simulink model "ACDCMG_woPV"  (R2022a)
settings: Solver=FixedStepAuto  StartTime=0.0  StopTime=0.2  FixedStep=Ts  MaxStep=1e-2  RelTol=1e-3
InitFcn:
  | Set_parameters_R2018
values from neighbouring files (symbols this model uses):
  D_invs = 0.05    [Set_parameters_R2018.m]
  dis11 = 3    [Set_parameters_R2018.m]
  dis14 = 2    [Set_parameters_R2018.m]
  dis2 = 0.2    [Set_parameters_R2018.m]
  dis3 = 0.15    [Set_parameters_R2018.m]
  dis4 = 0.4    [Set_parameters_R2018.m]
  dis5 = 0.4    [Set_parameters_R2018.m]
  dis6 = 0.4    [Set_parameters_R2018.m]
  dis8 = 2    [Set_parameters_R2018.m]
  Fnom = 60    [Set_parameters_R2018.m]
  H_invs = 6    [Set_parameters_R2018.m]
  max_min = 1    [Set_parameters_R2018.m]
  P_Load_3 = S_Load_3* PF_Load_3    (= 25500)    [Set_parameters_R2018.m]
  P_nom_inv = 3e3    (= 3000)    [Set_parameters_R2018.m]
  Pnom_T1 = 1.5e6    (= 1500000)    [Set_parameters_R2018.m]
  Pnom_T2 = 1.5e6    (= 1500000)    [Set_parameters_R2018.m]
  Pnom_T3 = 4e6    (= 4000000)    [Set_parameters_R2018.m]
  Ql_Load_3 = S_Load_3 * sin(acos(PF_Load_3))    [Set_parameters_R2018.m]
  R_Load_9 = (Vnom_prim * 1.35)^2 / P_Load_9    (= 1084.6153125)    [Set_parameters_R2018.m]
  R_Load_DC = Vnom_DC^2/ P_Load_DC    (= 45)    [Set_parameters_R2018.m]
  Rl = 0.394    [Set_parameters_R2018.m]
  Rls = 0.198    [Set_parameters_R2018.m]
  Ts = Ts_Power    (= 6.94444444444e-06)    [Set_parameters_R2018.m]
  Ts_Control = 6*Ts_Power    (= 4.16666666667e-05)    [Set_parameters_R2018.m]
  Ts_Power = 1/(24*Fnom)/100    (= 6.94444444444e-06)    [Set_parameters_R2018.m]
  V1_LL_T3 = 69e3    (= 69000)    [Set_parameters_R2018.m]
  Vnom_DC = 300    [Set_parameters_R2018.m]
  Vnom_Diesel = 2.4e3    (= 2400)    [Set_parameters_R2018.m]
  Vnom_prim = 13.8e3    (= 13800)    [Set_parameters_R2018.m]
  Vnom_sec = 220    [Set_parameters_R2018.m]
  Vnom_ter_AC_DC = 150    [Set_parameters_R2018.m]
  Xl = 0.1168    [Set_parameters_R2018.m]
  Xls = 0.1089    [Set_parameters_R2018.m]
undefined symbols (not defined in the file or in its folder): D1, Delta, DiscIntNeverNeededParam, ee_sli_rtmsupport, fn, gcbh, Ion, Lithium, S, sigbuilder_block, VnInv
libraries: powerlib_extras x55, spsCurrentMeasurementLib x53, powerlib_meascontrol x42, spsSeriesRLCBranchLib x32, spsVoltageMeasurementLib x31, spsRMSLib x29, spsThreePhaseVIMeasurementLib x24, simulink x21, spsThreePhaseSeriesRLCBranchLib x19, spsPower3phInstantaneousLib x15, spsPowerLib x12, spsGroundLib x11
(part 4 of 9)

== system ACDCMG_woPV/M1 ==
  Bus 9 Measurements : Scope  NumInputPorts=5
  Conv pu : Gain  Gain=sqrt (3)  SaturateOnIntegerOverflow=on  OutDataTypeStr=Inherit: Same as input  ParamDataTypeStr=Inherit: Same as input
  Conv pu1 : Gain  Gain=sqrt (3) /Vnom_prim  SaturateOnIntegerOverflow=on  OutDataTypeStr=Inherit: Same as input  ParamDataTypeStr=Inherit: Same as input
  "Power (3ph, Instantaneous)" : spsPower3phInstantaneousLib/Power (3ph, Instantaneous)
  Power Factor Block1 : Subsystem  mask(Power Factor Block){Freq=Fnom, Vinit=[0, 0], Iinit=[0, 0], Ts=0}
      mask prompts: Freq "Fundamental frequency (Hz):"; Vinit "Voltage initial input [ Mag, Phase (degrees) ]:"; Iinit "Current initial input [ Mag, Phase (degrees) ]:"; Ts "Sample time:"
      mask help:
      | Power Factor Block developed by Dr Rodney Tan
      | Version 1.01 (Aug 2016)
      |
      | Compute power factor and phase angle of AC circuit voltage-current pair at fundamental frequency.
      |
      | The computation is based on Power block and Complex number function block.
      |
      | For the first cycle of simulation, the outputs are held constant to the powers computed for the Voltage initial input and Current initial input parameters.
      mask Help:
      | <b>Fundamental Frequency (Hz)</b>
      | Specify the measurement fundamental frequency, in hertz, of the input signal.
      | 
      | <b>Voltage initial input [ Mag, Phase (degrees) ]</b>
      | Specify the voltage initial magnitude and phase to set a constant output for the first cycle of simulation.
      | 
      | <b>Current initial input [ Mag, Phase (degrees) ]</b>
      | Specify the current initial magnitude and phase to set a constant output for the first cycle of simulation.
      | 
      | <b>Sample Time</b>
      | Specify the sample time of the block, in seconds. Set to 0 to implement a continuous block.
      mask TypeOptions Freq: Power/Freq
      mask TypeOptions Vinit: Power/Vinit
      mask TypeOptions Iinit: Power/Iinit
      mask TypeOptions Ts: Power/Ts
  V L-L (rms) : Scope  NumInputPorts=2
  Vabc pu1 : Scope
  wires:
  Power Factor Block1/2("Iabc y Iabc ") -> Bus 9 Measurements/4
  Conv pu1/1 -> Vabc pu1/1
  Power Factor Block1/1("Vabc y Vabc ") -> Conv pu/1, Conv pu1/1, Bus 9 Measurements/3
  [IabcLL_Bus_9] -> "Power (3ph, Instantaneous)"/2, Power Factor Block1/2(Iabc)
  Conv pu/1 -> V L-L (rms)/1
  [Vab_bess] -> V L-L (rms)/2
  [VabcLL_Bus_9] -> "Power (3ph, Instantaneous)"/1, Power Factor Block1/1(Vabc)  "Vabc"
  "Power (3ph, Instantaneous)"/1 -> Bus 9 Measurements/1
  "Power (3ph, Instantaneous)"/2 -> Bus 9 Measurements/2
  Power Factor Block1/3(Outport) -> Bus 9 Measurements/5

== system ACDCMG_woPV/M2 ==
  Bus 1 Measurement : Scope  NumInputPorts=4
  Conv pu : Gain  Gain=sqrt (3)  SaturateOnIntegerOverflow=on  OutDataTypeStr=Inherit: Same as input  ParamDataTypeStr=Inherit: Same as input
  Conv pu1 : Gain  Gain=sqrt (3) /Vnom_sec  SaturateOnIntegerOverflow=on  OutDataTypeStr=Inherit: Same as input  ParamDataTypeStr=Inherit: Same as input
  "Power (3ph, Instantaneous)" : spsPower3phInstantaneousLib/Power (3ph, Instantaneous)
  Power Factor Block1 : Subsystem  mask(Power Factor Block){Freq=Fnom, Vinit=[0, 0], Iinit=[0, 0], Ts=0}
      mask prompts: Freq "Fundamental frequency (Hz):"; Vinit "Voltage initial input [ Mag, Phase (degrees) ]:"; Iinit "Current initial input [ Mag, Phase (degrees) ]:"; Ts "Sample time:"
      mask help:
      | Power Factor Block developed by Dr Rodney Tan
      | Version 1.01 (Aug 2016)
      |
      | Compute power factor and phase angle of AC circuit voltage-current pair at fundamental frequency.
      |
      | The computation is based on Power block and Complex number function block.
      |
      | For the first cycle of simulation, the outputs are held constant to the powers computed for the Voltage initial input and Current initial input parameters.
      mask Help:
      | <b>Fundamental Frequency (Hz)</b>
      | Specify the measurement fundamental frequency, in hertz, of the input signal.
      | 
      | <b>Voltage initial input [ Mag, Phase (degrees) ]</b>
      | Specify the voltage initial magnitude and phase to set a constant output for the first cycle of simulation.
      | 
      | <b>Current initial input [ Mag, Phase (degrees) ]</b>
      | Specify the current initial magnitude and phase to set a constant output for the first cycle of simulation.
      | 
      | <b>Sample Time</b>
      | Specify the sample time of the block, in seconds. Set to 0 to implement a continuous block.
      mask TypeOptions Freq: Power/Freq
      mask TypeOptions Vinit: Power/Vinit
      mask TypeOptions Iinit: Power/Iinit
      mask TypeOptions Ts: Power/Ts
  V L-L (rms) : Scope  NumInputPorts=2
  Vabc pu1 : Scope
  wires:
  Power Factor Block1/2("Iabc y Iabc ") -> Bus 1 Measurement/4
  Conv pu1/1 -> Vabc pu1/1
  Power Factor Block1/1("Vabc y Vabc ") -> Conv pu/1, Conv pu1/1, Bus 1 Measurement/3
  [IabcLL_Bus_1] -> "Power (3ph, Instantaneous)"/2, Power Factor Block1/2(Iabc)
  Conv pu/1 -> V L-L (rms)/1
  [Vab_bess] -> V L-L (rms)/2
  [VabcLL_Bus_1] -> "Power (3ph, Instantaneous)"/1, Power Factor Block1/1(Vabc)  "Vabc"
  "Power (3ph, Instantaneous)"/1 -> Bus 1 Measurement/1
  "Power (3ph, Instantaneous)"/2 -> Bus 1 Measurement/2

== system ACDCMG_woPV/M4 ==
  Bus 6 Measurements : Scope  NumInputPorts=4
  Conv pu1 : Gain  Gain=sqrt (3) /Vnom_prim  SaturateOnIntegerOverflow=on  OutDataTypeStr=Inherit: Same as input  ParamDataTypeStr=Inherit: Same as input
  "Power (3ph, Instantaneous)" : spsPower3phInstantaneousLib/Power (3ph, Instantaneous)
  Power Factor Block1 : Subsystem  mask(Power Factor Block){Freq=Fnom, Vinit=[0, 0], Iinit=[0, 0], Ts=0}
      mask prompts: Freq "Fundamental frequency (Hz):"; Vinit "Voltage initial input [ Mag, Phase (degrees) ]:"; Iinit "Current initial input [ Mag, Phase (degrees) ]:"; Ts "Sample time:"
      mask help:
      | Power Factor Block developed by Dr Rodney Tan
      | Version 1.01 (Aug 2016)
      |
      | Compute power factor and phase angle of AC circuit voltage-current pair at fundamental frequency.
      |
      | The computation is based on Power block and Complex number function block.
      |
      | For the first cycle of simulation, the outputs are held constant to the powers computed for the Voltage initial input and Current initial input parameters.
      mask Help:
      | <b>Fundamental Frequency (Hz)</b>
      | Specify the measurement fundamental frequency, in hertz, of the input signal.
      | 
      | <b>Voltage initial input [ Mag, Phase (degrees) ]</b>
      | Specify the voltage initial magnitude and phase to set a constant output for the first cycle of simulation.
      | 
      | <b>Current initial input [ Mag, Phase (degrees) ]</b>
      | Specify the current initial magnitude and phase to set a constant output for the first cycle of simulation.
      | 
      | <b>Sample Time</b>
      | Specify the sample time of the block, in seconds. Set to 0 to implement a continuous block.
      mask TypeOptions Freq: Power/Freq
      mask TypeOptions Vinit: Power/Vinit
      mask TypeOptions Iinit: Power/Iinit
      mask TypeOptions Ts: Power/Ts
  Vabc pu1 : Scope
  wires:
  [IabcLL_Bus_6] -> "Power (3ph, Instantaneous)"/2, Power Factor Block1/2(Iabc)
  Power Factor Block1/2("Iabc y Iabc ") -> Bus 6 Measurements/4
  Conv pu1/1 -> Vabc pu1/1
  Power Factor Block1/1("Vabc y Vabc ") -> Conv pu1/1, Bus 6 Measurements/3
  [VabcLL_Bus_6] -> "Power (3ph, Instantaneous)"/1, Power Factor Block1/1(Vabc)  "Signal Vabc"
  "Power (3ph, Instantaneous)"/1 -> Bus 6 Measurements/1
  "Power (3ph, Instantaneous)"/2 -> Bus 6 Measurements/2

== system ACDCMG_woPV/Main Grid 69 kV Inf ==
  note: Thevenin equivalent
  Ground1 : spsGroundLib/Ground  LConnTagsString=a
  Programmable Voltage Source1 : spsThreePhaseProgrammableVoltageSourceLib/Three-Phase Programmable Voltage Source  PositiveSequence="[69e3 0  60]"  VariationEntity=None  VariationType=Table of time-amplitude pairs  VariationTypeAlt=Step  VariationStep=-0.3  VariationRate=0.5  VariationMagnitude=0.4  VariationFrequency=2  VariationTiming=[0.1 1.2]  VariationPhaseA=off  Amplitudes=[1]  TimeValues=[0]  HarmonicGeneration=off  HarmonicA=[3 0.2 -25 0]  HarmonicB="[2 0.15  35 2]"  Timing="[0.1  0.6]"  BusType=swing  Pref=500  Qref=0  Qmin=-inf  Qmax=inf
  C : PMIOPort  Side=Right
  B : PMIOPort  Port=2  Side=Right
  A : PMIOPort  Port=3  Side=Right
  connections:
  C/RConn1 -- Programmable Voltage Source1/RConn3
  Ground1/LConn1 -- Programmable Voltage Source1/LConn1
  B/RConn1 -- Programmable Voltage Source1/RConn2
  A/RConn1 -- Programmable Voltage Source1/RConn1

== system ACDCMG_woPV/Non Linear AC  Load 9 ==
  Display : Display
  Mean : powerlib_meascontrol/Measurements/Mean  Freq=100  Vinit=0  Ts=0
  No lineal AC Load 320Kw : spsUniversalBridgeLib/Universal Bridge  Arms=3  SnubberResistance=1e5  SnubberCapacitance=inf  Device=Thyristors  Ron=1e-3  Lon=0  ForwardVoltages="[  0  0  ]"  ForwardVoltage=0  GTOparameters=[ 10e-6 , 20e-6 ]  IGBTparameters=[ 1e-6 , 2e-6 ]  Measurements=None  Measurements_2=None  converterType=Rectifier
  PWM Generator (2-Level) : powerlib_meascontrol/Pulse & Signal Generators/PWM Generator (2-Level)  ModulatorType=Three-phase bridge (6 pulses)  ModulatorMode=Unsynchronized  Fc=4080  Pc=0  nF=27  MinMax="[ -1  1 ]"  SamplingTechnique=Natural  ModulatingSignals=on  m=0.8  Freq=Fnom  Phase=-30  Ts=0  ShowCarrierOutport=off
  RL : spsSeriesRLCBranchLib/Series RLC Branch  LConnTagsString=__new0  RConnTagsString=__new0  BranchType=R  Resistance=R_Load_9  Inductance=5e-3  SetiL0=off  InitialCurrent=0  Capacitance=1e-6  Setx0=off  InitialVoltage=0  Measurements=None
  RL1 : spsSeriesRLCBranchLib/Series RLC Branch  LConnTagsString=__new0  RConnTagsString=__new0  BranchType=C  Resistance=1  Inductance=5e-3  SetiL0=off  InitialCurrent=0  Capacitance=10e-6  Setx0=off  InitialVoltage=0  Measurements=None
  "Vdc " : spsVoltageMeasurementLib/Voltage Measurement  Tag=PoWeRsYsTeMmEaSuReMeNt  PhasorSimulation=off  OutputType=Magnitude  PSBequivalent=0
  A : PMIOPort  Tag=PMCPort  Side=Left
  B : PMIOPort  Tag=PMCPort  Port=2  Side=Left
  C : PMIOPort  Tag=PMCPort  Port=3  Side=Left
  wires:
  PWM Generator (2-Level)/1 -> No lineal AC Load 320Kw/1
  "Vdc "/1 -> Mean/1
  Mean/1 -> Display/1
  connections:
  No lineal AC Load 320Kw/RConn1 -- "Vdc "/LConn1 -- RL1/LConn1 -- RL/LConn1
  A/RConn1 -- No lineal AC Load 320Kw/LConn1
  C/RConn1 -- No lineal AC Load 320Kw/LConn3
  B/RConn1 -- No lineal AC Load 320Kw/LConn2
  No lineal AC Load 320Kw/RConn2 -- "Vdc "/LConn2 -- RL1/RConn1 -- RL/RConn1

== system ACDCMG_woPV/Resource1 ==
  note: http://calculationsolar.com/blog/?cat=2
  Constant1 : Constant  Value=max_min
  Irradiance (W/m^2) : Display
      settings: Format=bank  Decimation=1000
  Irradiance Temp Demand Max : Subsystem  Tag=STV Subsys  LoadFcn=sigbuilder_block('load');  StartFcn=sigbuilder_block('start');  StopFcn=sigbuilder_block('stop');  ClipboardFcn=sigbuilder_block('clipboard');  mask(Sigbuilder block){tuvar=[0:10]}
      mask help: Sigbuilder GUI
      mask init:
      | if ~strcmp(get_param(bdroot(gcbh),'SimulationStatus'),'stopped') tuvar = sigbuilder_block('maskInit'); end
      settings: CopyFcn=sigbuilder_block('copy');  DeleteFcn=sigbuilder_block('delete');  ModelCloseFcn=sigbuilder_block('modelClose');  PreSaveFcn=sigbuilder_block('preSave');  PauseFcn=sigbuilder_block('pause')  ContinueFcn=sigbuilder_block('continue')  NameChangeFcn=sigbuilder_block('namechange');  OpenFcn=sigbuilder_block('open',[0 30 1024.5 488.25 ]);  CloseFcn=sigbuilder_block('close');
      mask Display: plot(0, 0, 100, 100,[2, 2, 32, 32, 2], [68, 8, 8, 68, 68],[32, 2], [38, 38], [32, 19, 2],[53, 60, 44], [32, 17, 17, 2],[16, 16, 31, 31]);txt = getActiveGroup(gcbh);text(2, 100, txt,'verticalAlignment', 'top');
  Irradiance MIn Demand : Constant  Value=0
  Switch2 : Switch  Criteria=u2 > Threshold  SaturateOnIntegerOverflow=off  InputSameDT=off
  Temperature (deg. C) : Display
      settings: Format=bank  Decimation=1000
  Temp : Outport  VectorParamsAs1DForOutWhenUnconnected=off
  Ir : Outport  Port=2  VectorParamsAs1DForOutWhenUnconnected=off
  wires:
  Irradiance Temp Demand Max/1(Ir) -> Switch2/1, Irradiance (W/m^2)/1
  Irradiance Temp Demand Max/2(Temp) -> Temp/1, Temperature (deg. C)/1
  Irradiance MIn Demand/1 -> Switch2/3
  Constant1/1 -> Switch2/2
  Switch2/1 -> Ir/1  "Radiación (kW/m2)"

== system ACDCMG_woPV/Smart Meter: Grid  ==
  Bus 3 Measurements : Scope  NumInputPorts=4
  Conv pu1 : Gain  Gain=sqrt (3) /Vnom_prim  SaturateOnIntegerOverflow=on  OutDataTypeStr=Inherit: Same as input  ParamDataTypeStr=Inherit: Same as input
  "Power (3ph, Instantaneous)" : spsPower3phInstantaneousLib/Power (3ph, Instantaneous)
  Power Factor Block1 : Subsystem  mask(Power Factor Block){Freq=Fnom, Vinit=[0, 0], Iinit=[0, 0], Ts=0}
      mask prompts: Freq "Fundamental frequency (Hz):"; Vinit "Voltage initial input [ Mag, Phase (degrees) ]:"; Iinit "Current initial input [ Mag, Phase (degrees) ]:"; Ts "Sample time:"
      mask help:
      | Power Factor Block developed by Dr Rodney Tan
      | Version 1.01 (Aug 2016)
      |
      | Compute power factor and phase angle of AC circuit voltage-current pair at fundamental frequency.
      |
      | The computation is based on Power block and Complex number function block.
      |
      | For the first cycle of simulation, the outputs are held constant to the powers computed for the Voltage initial input and Current initial input parameters.
      mask Help:
      | <b>Fundamental Frequency (Hz)</b>
      | Specify the measurement fundamental frequency, in hertz, of the input signal.
      | 
      | <b>Voltage initial input [ Mag, Phase (degrees) ]</b>
      | Specify the voltage initial magnitude and phase to set a constant output for the first cycle of simulation.
      | 
      | <b>Current initial input [ Mag, Phase (degrees) ]</b>
      | Specify the current initial magnitude and phase to set a constant output for the first cycle of simulation.
      | 
      | <b>Sample Time</b>
      | Specify the sample time of the block, in seconds. Set to 0 to implement a continuous block.
      mask TypeOptions Freq: Power/Freq
      mask TypeOptions Vinit: Power/Vinit
      mask TypeOptions Iinit: Power/Iinit
      mask TypeOptions Ts: Power/Ts
  Vabc pu1 : Scope
  wires:
  [Iabc_LL_Bus3] -> "Power (3ph, Instantaneous)"/2, Power Factor Block1/2(Iabc)  "Signal Iabc"
  Power Factor Block1/2("Iabc y Iabc ") -> Bus 3 Measurements/4
  Conv pu1/1 -> Vabc pu1/1
  Power Factor Block1/1("Vabc y Vabc ") -> Conv pu1/1, Bus 3 Measurements/3
  [Vabc_LL_Bus3] -> "Power (3ph, Instantaneous)"/1, Power Factor Block1/1(Vabc)  "Vabc"
  "Power (3ph, Instantaneous)"/1 -> Bus 3 Measurements/1
  "Power (3ph, Instantaneous)"/2 -> Bus 3 Measurements/2

== system ACDCMG_woPV/Smart Meter: Unbalanced Load ==
  Conv pu1 : Gain  Gain=sqrt (3) /Vnom_sec  SaturateOnIntegerOverflow=on  OutDataTypeStr=Inherit: Same as input  ParamDataTypeStr=Inherit: Same as input
  Measurement1 : Scope  NumInputPorts=4
  "Power (3ph, Instantaneous)" : spsPower3phInstantaneousLib/Power (3ph, Instantaneous)
  Power Factor Block1 : Subsystem  mask(Power Factor Block){Freq=Fnom, Vinit=[0, 0], Iinit=[0, 0], Ts=0}
      mask prompts: Freq "Fundamental frequency (Hz):"; Vinit "Voltage initial input [ Mag, Phase (degrees) ]:"; Iinit "Current initial input [ Mag, Phase (degrees) ]:"; Ts "Sample time:"
      mask help:
      | Power Factor Block developed by Dr Rodney Tan
      | Version 1.01 (Aug 2016)
      |
      | Compute power factor and phase angle of AC circuit voltage-current pair at fundamental frequency.
      |
      | The computation is based on Power block and Complex number function block.
      |
      | For the first cycle of simulation, the outputs are held constant to the powers computed for the Voltage initial input and Current initial input parameters.
      mask Help:
      | <b>Fundamental Frequency (Hz)</b>
      | Specify the measurement fundamental frequency, in hertz, of the input signal.
      | 
      | <b>Voltage initial input [ Mag, Phase (degrees) ]</b>
      | Specify the voltage initial magnitude and phase to set a constant output for the first cycle of simulation.
      | 
      | <b>Current initial input [ Mag, Phase (degrees) ]</b>
      | Specify the current initial magnitude and phase to set a constant output for the first cycle of simulation.
      | 
      | <b>Sample Time</b>
      | Specify the sample time of the block, in seconds. Set to 0 to implement a continuous block.
      mask TypeOptions Freq: Power/Freq
      mask TypeOptions Vinit: Power/Vinit
      mask TypeOptions Iinit: Power/Iinit
      mask TypeOptions Ts: Power/Ts
  Vabc pu1 : Scope
  wires:
  [Iabc_load_2] -> "Power (3ph, Instantaneous)"/2, Power Factor Block1/2(Iabc)
  [Vabc_load_2] -> "Power (3ph, Instantaneous)"/1, Power Factor Block1/1(Vabc)  "Signal Vabc"
  Power Factor Block1/2("Iabc y Iabc ") -> Measurement1/4
  Conv pu1/1 -> Vabc pu1/1
  Power Factor Block1/1(Vabc y Vabc) -> Conv pu1/1, Measurement1/3
  "Power (3ph, Instantaneous)"/1 -> Measurement1/1
  "Power (3ph, Instantaneous)"/2 -> Measurement1/2

== system ACDCMG_woPV/Boost -buck Bi-directional converter 1 0.65 kW/+ve reference For Buck --> -ve reference For Boost <-- ==
  note: Buck PWM
  note: Duty Cycle
  note: Upper logic
  note: Lower logic
  note: Boost PWM
  note: Duty Cycle
  I_ref : Inport
  PID Orig Boost : Subsystem
  PID Orig Buck : Subsystem
  Relational Operator : RelationalOperator  Operator=>  OutDataTypeStr=boolean  InputSameDT=off
  Relational Operator1 : RelationalOperator  Operator=>  OutDataTypeStr=boolean  InputSameDT=off
  Saturation : Saturate  UpperLimit=0.9  LowerLimit=0
  Saturation1 : Saturate  UpperLimit=0.8  LowerLimit=0
  Sawtooth : simulink/Sources/Repeating Sequence  rep_seq_t=[0 1/5000]  rep_seq_y=[0 1]
  Sawtooth1 : simulink/Sources/Repeating Sequence  rep_seq_t=[0 1/5000]  rep_seq_y=[0 1]
  Sign : Gain  Gain=-1
  Sign1 : Gain  Gain=-1
  Sum : Sum  Inputs=|+-
  Sum2 : Sum  Inputs=-+|
  Switch : Switch  Criteria=u2 > Threshold  SaturateOnIntegerOverflow=off  InputSameDT=off
  Switch1 : Switch  SaturateOnIntegerOverflow=off  InputSameDT=off
  Vref1 : Constant  Value=0
  Vref2 : Constant  Value=0
  buck_I_Ctrl : Outport  VectorParamsAs1DForOutWhenUnconnected=off
  boost_I_Ctrl : Outport  Port=2  VectorParamsAs1DForOutWhenUnconnected=off
  wires:
  Sum/1 -> PID Orig Boost/1(error)  "error"
  Relational Operator/1 -> [boost1]
  Sign/1 -> Sum/1
  PID Orig Boost/1(Out1) -> Saturation/1
  PID Orig Buck/1(Out1) -> Saturation1/1
  Sawtooth/1 -> Relational Operator/2
  Sawtooth1/1 -> Relational Operator1/2
  Relational Operator1/1 -> [buck1]
  Sum2/1 -> PID Orig Buck/1(error)  "error"
  Saturation/1 -> Relational Operator/1
  Saturation1/1 -> Relational Operator1/1
  Vref1/1 -> Switch/3
  Vref2/1 -> Switch1/1
  [boost1] -> Switch1/3
  [buck1] -> Switch/1
  I_ref/1 -> Switch1/2, Switch/2, Sum2/2, Sign/1  "Current Reference"
  Sign1/1 -> Sum/2
  Switch1/1 -> boost_I_Ctrl/1
  Switch/1 -> buck_I_Ctrl/1
  [current] -> Sum2/1, Sign1/1

== system ACDCMG_woPV/Boost -buck Bi-directional converter 1 0.65 kW/OP_max // min ==
  boost_V_Ctrll : Inport
  buck_V_Ctrl : Inport  Port=2
  buck_I_Ctrl : Inport  Port=3
  boost_I_Ctrll : Inport  Port=4
  Control modes 0- Current 1- Coltage : Constant
  OP_max1 : Constant
  OP_min1 : Constant  Value=0
  Switch1 : Switch  Criteria=u2 > Threshold  SaturateOnIntegerOverflow=off  InputSameDT=off
  Switch2 : Switch  Criteria=u2 > Threshold  SaturateOnIntegerOverflow=off  InputSameDT=off
  Switch3 : Switch  Criteria=u2 > Threshold  SaturateOnIntegerOverflow=off  InputSameDT=off
  Op_Max / Min : Outport  VectorParamsAs1DForOutWhenUnconnected=off
  g_buck : Outport  Port=2  VectorParamsAs1DForOutWhenUnconnected=off
  g_boost : Outport  Port=3  VectorParamsAs1DForOutWhenUnconnected=off
  wires:
  OP_max1/1 -> Switch2/1
  OP_min1/1 -> Switch2/3
  Switch2/1 -> Op_Max / Min/1
  Control modes 0- Current 1- Coltage/1 -> Switch2/2, Switch1/2, Switch3/2
  boost_I_Ctrll/1 -> Switch1/3
  boost_V_Ctrll/1 -> Switch1/1
  buck_V_Ctrl/1 -> Switch3/1
  buck_I_Ctrl/1 -> Switch3/3
  Switch1/1 -> g_boost/1
  Switch3/1 -> g_buck/1

== system ACDCMG_woPV/Boost -buck Bi-directional converter 1 0.65 kW/Primary Control ==
  V_ref : Inport
  Constant : Constant
  Display3 : Display  Commented=on
  From1 : From  Commented=on  GotoTag=Vdc_bus  TagVisibility=global
  From4 : From  Commented=on  GotoTag=boost1
  From5 : From  Commented=on  GotoTag=buck1
  PID Orig Boost : Subsystem
  Relational Operator2 : RelationalOperator  Commented=on  Operator=>  OutDataTypeStr=boolean  InputSameDT=off
  Saturation : Saturate  UpperLimit=0.9  LowerLimit=0.1
  Scope1 : Scope
  Sum : Sum  Inputs=|+-
  Sum1 : Sum  Inputs=|-+
  Switch : Switch  Commented=on  Criteria=u2 > Threshold  Threshold=300  SaturateOnIntegerOverflow=off  InputSameDT=off
  Switch1 : Switch  Commented=on  Criteria=u2 > Threshold  Threshold=300  SaturateOnIntegerOverflow=off  InputSameDT=off
  Vref1 : Constant  Commented=on  Value=0
  Vref2 : Constant  Commented=on  Value=0
  Duty_Ctrl : Outport  VectorParamsAs1DForOutWhenUnconnected=off
  Comp_Duty_Ctrl : Outport  Port=2  VectorParamsAs1DForOutWhenUnconnected=off
  wires:
  Relational Operator2/1 -> Switch1/2, Switch/2
  V_ref/1 -> Sum/1, Relational Operator2/2
  From1/1 -> Relational Operator2/1
  Vref2/1 -> Switch1/1
  [Vdc_bus] -> Sum/2
  From5/1 -> Switch/1
  From4/1 -> Switch1/3
  Switch/1 -> Display3/1
  Vref1/1 -> Switch/3
  Sum/1 -> PID Orig Boost/1(error)  "error"
  PID Orig Boost/1(Out1) -> Saturation/1
  Constant/1 -> Sum1/2
  Saturation/1 -> Sum1/1, Duty_Ctrl/1, Scope1/1
  Sum1/1 -> Comp_Duty_Ctrl/1

== system ACDCMG_woPV/Boost -buck Bi-directional converter DC //CD 1 0.65 kW/+ve reference For Buck --> -ve reference For Boost <-- ==
  note: Notes :
      | 1- Saturation block : in practical applications during experiment, in the begining if the experiment, the error is usually high, therefore, duty cycle might reach value of 1, which means the IGBT switch will be shorted for a while which might cause damage to your circuit. it is preferable to put the saturation value to 0.7 during experiment, once you trust your circuit, you can increase up to 0.9.
      | 2- Sawtooth : We choose the frequancy of the sawtooth to be 5 kHz, because according to some papers if you go beyond this value, parastic elements will show up (i.e. its like an imaginary resistance and capcitance that causes switching losses and heat). But the more you increase the frequency, the smoother the signal you will get.
      | 3- Step size of your mode l: Make sure that the step size (sample time) in the "model configuration parameters" is smaller than 1/f of the sawtooth. For example, lets say that the sawtooth f = 2 Hz or cycle/sec, meaning the triangle (cycle) repeats every 1/2 sec. Step size or sample time means how many point matlab plot every cycle, lets say it is 1/4 (i.e. plot a point every 0.25 sec), that means that the triangle will be plotted with only two points. That reduce the accuracy, Moreover if the step size is greater than 1/f of the sawtooth, the sawtooth output will be zero.
  note: Buck PWM
  note: Duty Cycle
  note: Upper logic
  note: Lower logic
  note: Boost PWM
  note: Duty Cycle
  I_ref : Inport
  Display3 : Display
  Display4 : Display
  Integrator : Integrator  LimitOutput=on  UpperSaturationLimit=0.9  LowerSaturationLimit=0
  Integrator1 : Integrator  LimitOutput=on  UpperSaturationLimit=0.9  LowerSaturationLimit=0
  Ki : Gain  Gain=3
  Ki1 : Gain  Gain=110
  Kp : Gain  Gain=0.02
  Kp1 : Gain  Gain=0.2
  Relational Operator : RelationalOperator  Operator=>  OutDataTypeStr=boolean  InputSameDT=off
  Relational Operator1 : RelationalOperator  Operator=>  OutDataTypeStr=boolean  InputSameDT=off
  Saturation : Saturate  UpperLimit=0.9  LowerLimit=0
  Saturation1 : Saturate  UpperLimit=0.8  LowerLimit=0
  Sawtooth : simulink/Sources/Repeating Sequence  rep_seq_t=[0 1/5000]  rep_seq_y=[0 1]
  Sawtooth1 : simulink/Sources/Repeating Sequence  rep_seq_t=[0 1/5000]  rep_seq_y=[0 1]
  Sign : Gain  Gain=-1
  Sign1 : Gain  Gain=-1
  Sum : Sum  Inputs=|+-
  Sum1 : Sum  Inputs=|++
  Sum2 : Sum  Inputs=|+-
  Sum3 : Sum  Inputs=|++
  Switch : Switch  Criteria=u2 > Threshold  SaturateOnIntegerOverflow=off  InputSameDT=off
  Switch1 : Switch  SaturateOnIntegerOverflow=off  InputSameDT=off
  Vref1 : Constant  Value=0
  Vref2 : Constant  Value=0
  buck : Outport  VectorParamsAs1DForOutWhenUnconnected=off
  boost : Outport  Port=2  VectorParamsAs1DForOutWhenUnconnected=off
  tag scope: boost1=global, buck1=global
  wires:
  Integrator/1 -> Sum1/2
  Kp/1 -> Sum1/1
  Sum/1 -> Kp/1, Ki/1  "error"
  Relational Operator/1 -> [boost1]
  Sign/1 -> Sum/1
  Sum1/1 -> Saturation/1
  Ki/1 -> Integrator/1
  Sum3/1 -> Saturation1/1
  Integrator1/1 -> Sum3/2
  Sawtooth/1 -> Relational Operator/2
  Sawtooth1/1 -> Relational Operator1/2
  [current] -> Sum2/2, Sign1/1
  Kp1/1 -> Sum3/1
  Relational Operator1/1 -> [buck1]
  Sum2/1 -> Ki1/1, Kp1/1  "error"
  Saturation/1 -> Relational Operator/1
  Saturation1/1 -> Relational Operator1/1
  Ki1/1 -> Integrator1/1
  Vref1/1 -> Switch/3
  Vref2/1 -> Switch1/1
  [boost1] -> Switch1/3
  [buck1] -> Switch/1
  I_ref/1 -> Sum2/1, Sign/1, Switch1/2, Switch/2  "Current Reference"
  Sign1/1 -> Sum/2
  Switch1/1 -> Display4/1, boost/1
  Switch/1 -> Display3/1, buck/1

== system ACDCMG_woPV/Boost -buck Bi-directional converter DC //CD 1 0.65 kW/ref ==
  note: 1 -charge
      | 0-discharge
  Constant2 : Constant  Value=max_min
  Constant3 : Constant  Value=max_min
  Current reference (battery charge) OP_Max : Constant  Value=5
  Current reference (battery discharge) OP_Max1 : Constant  Value=-5
  Min Demand OP_min : Constant  Value=3
  Min Demand OP_min1 : Constant  Value=-3
  Switch : Switch  Criteria=u2 > Threshold  SaturateOnIntegerOverflow=off  InputSameDT=off
  Switch1 : Switch  Criteria=u2 > Threshold  SaturateOnIntegerOverflow=off  InputSameDT=off
  Switch3 : Switch  Criteria=u2 > Threshold  SaturateOnIntegerOverflow=off  InputSameDT=off
  Vref1 : Constant
  ref : Outport  VectorParamsAs1DForOutWhenUnconnected=off
  wires:
  Constant3/1 -> Switch3/2
  Switch3/1 -> Switch/3
  Switch1/1 -> Switch/1
  Vref1/1 -> Switch/2
  Min Demand OP_min/1 -> Switch1/3
  Current reference (battery charge) OP_Max/1 -> Switch1/1
  Min Demand OP_min1/1 -> Switch3/3
  Constant2/1 -> Switch1/2
  Current reference (battery discharge) OP_Max1/1 -> Switch3/1
  Switch/1 -> ref/1

== system ACDCMG_woPV/Boost -buck Bi-directional converter DC //DC 1 0.65 kW Switching Model/+ve reference For Buck --> -ve reference For Boost <-- ==
  note: Buck PWM
  note: Duty Cycle
  note: Upper logic
  note: Lower logic
  note: Boost PWM
  note: Duty Cycle
  I_ref : Inport
  PID Orig Boost : Subsystem
  PID Orig Buck : Subsystem
  Relational Operator : RelationalOperator  Operator=>  OutDataTypeStr=boolean  InputSameDT=off
  Relational Operator1 : RelationalOperator  Operator=>  OutDataTypeStr=boolean  InputSameDT=off
  Saturation : Saturate  UpperLimit=0.9  LowerLimit=0
  Saturation1 : Saturate  UpperLimit=0.8  LowerLimit=0
  Sawtooth : simulink/Sources/Repeating Sequence  rep_seq_t=[0 1/5000]  rep_seq_y=[0 1]
  Sawtooth1 : simulink/Sources/Repeating Sequence  rep_seq_t=[0 1/5000]  rep_seq_y=[0 1]
  Sign : Gain  Gain=-1
  Sign1 : Gain  Gain=-1
  Sum : Sum  Inputs=|+-
  Sum2 : Sum  Inputs=-+|
  Switch : Switch  Criteria=u2 > Threshold  SaturateOnIntegerOverflow=off  InputSameDT=off
  Switch1 : Switch  SaturateOnIntegerOverflow=off  InputSameDT=off
  Vref1 : Constant  Value=0
  Vref2 : Constant  Value=0
  buck_I_Ctrl : Outport  VectorParamsAs1DForOutWhenUnconnected=off
  boost_I_Ctrl : Outport  Port=2  VectorParamsAs1DForOutWhenUnconnected=off
  wires:
  Sum/1 -> PID Orig Boost/1(error)  "error"
  Relational Operator/1 -> [boost1]
  Sign/1 -> Sum/1
  PID Orig Boost/1(Out1) -> Saturation/1
  PID Orig Buck/1(Out1) -> Saturation1/1
  Sawtooth/1 -> Relational Operator/2
  Sawtooth1/1 -> Relational Operator1/2
  Relational Operator1/1 -> [buck1]
  Sum2/1 -> PID Orig Buck/1(error)  "error"
  Saturation/1 -> Relational Operator/1
  Saturation1/1 -> Relational Operator1/1
  Vref1/1 -> Switch/3
  Vref2/1 -> Switch1/1
  [boost1] -> Switch1/3
  [buck1] -> Switch/1
  I_ref/1 -> Switch1/2, Switch/2, Sum2/2, Sign/1  "Current Reference"
  Sign1/1 -> Sum/2
  Switch1/1 -> boost_I_Ctrl/1
  Switch/1 -> buck_I_Ctrl/1
  [current] -> Sum2/1, Sign1/1

== system ACDCMG_woPV/Boost -buck Bi-directional converter DC //DC 1 0.65 kW Switching Model/OP_max // min ==
  boost_V_Ctrll : Inport
  buck_V_Ctrl : Inport  Port=2
  buck_I_Ctrl : Inport  Port=3
  boost_I_Ctrll : Inport  Port=4
  Control modes 0- Current 1- Coltage : Constant
  OP_max1 : Constant
  OP_min1 : Constant  Value=0
  Switch1 : Switch  Criteria=u2 > Threshold  SaturateOnIntegerOverflow=off  InputSameDT=off
  Switch2 : Switch  Criteria=u2 > Threshold  SaturateOnIntegerOverflow=off  InputSameDT=off
  Switch3 : Switch  Criteria=u2 > Threshold  SaturateOnIntegerOverflow=off  InputSameDT=off
  Op_Max / Min : Outport  VectorParamsAs1DForOutWhenUnconnected=off
  g_buck : Outport  Port=2  VectorParamsAs1DForOutWhenUnconnected=off
  g_boost : Outport  Port=3  VectorParamsAs1DForOutWhenUnconnected=off
  wires:
  OP_max1/1 -> Switch2/1
  OP_min1/1 -> Switch2/3
  Switch2/1 -> Op_Max / Min/1
  Control modes 0- Current 1- Coltage/1 -> Switch2/2, Switch1/2, Switch3/2
  boost_I_Ctrll/1 -> Switch1/3
  boost_V_Ctrll/1 -> Switch1/1
  buck_V_Ctrl/1 -> Switch3/1
  buck_I_Ctrl/1 -> Switch3/3
  Switch1/1 -> g_boost/1
  Switch3/1 -> g_buck/1

== system ACDCMG_woPV/Boost -buck Bi-directional converter DC //DC 1 0.65 kW Switching Model/Primary Control ==
  V_ref : Inport
  Display3 : Display
  Display4 : Display
  PID Orig Boost : Subsystem
  PID Orig Buck : Subsystem
  Relational Operator : RelationalOperator  Operator=>  OutDataTypeStr=boolean  InputSameDT=off
  Relational Operator1 : RelationalOperator  Operator=>  OutDataTypeStr=boolean  InputSameDT=off
  Relational Operator2 : RelationalOperator  Operator=>  OutDataTypeStr=boolean  InputSameDT=off
  Repeating Sequence : simulink/Sources/Repeating Sequence  rep_seq_t=[0 1/5000]  rep_seq_y=[0 1]
  Repeating Sequence1 : simulink/Sources/Repeating Sequence  rep_seq_t=[0 1/5000]  rep_seq_y=[0 1]
  Saturation : Saturate  UpperLimit=0.9  LowerLimit=0
  Saturation1 : Saturate  UpperLimit=0.9  LowerLimit=0
  Sum : Sum  Inputs=|+-
  Sum2 : Sum  Inputs=|+-
  Switch : Switch  Criteria=u2 > Threshold  Threshold=300  SaturateOnIntegerOverflow=off  InputSameDT=off
  Switch1 : Switch  Criteria=u2 > Threshold  Threshold=300  SaturateOnIntegerOverflow=off  InputSameDT=off
  Vref1 : Constant  Value=0
  Vref2 : Constant  Value=0
  buck_V_Ctrl : Outport  VectorParamsAs1DForOutWhenUnconnected=off
  boost_V_Ctrl : Outport  Port=2  VectorParamsAs1DForOutWhenUnconnected=off
  wires:
  Relational Operator2/1 -> Switch1/2, Switch/2
  Saturation1/1 -> Relational Operator1/1
  V_ref/1 -> Sum/1, Relational Operator2/2, Sum2/1
  [Vdc_bus] -> Relational Operator2/1
  Vref2/1 -> Switch1/1
  Repeating Sequence/1 -> Relational Operator/2
  Repeating Sequence1/1 -> Relational Operator1/2
  Relational Operator1/1 -> [buck1]
  [Vdc_bus] -> Sum2/2, Sum/2
  [buck1] -> Switch/1
  Switch1/1 -> Display4/1, boost_V_Ctrl/1
  Saturation/1 -> Relational Operator/1
  [boost1] -> Switch1/3
  Sum2/1 -> PID Orig Buck/1(error)  "error"
  Relational Operator/1 -> [boost1]
  Switch/1 -> Display3/1, buck_V_Ctrl/1
  Vref1/1 -> Switch/3
  Sum/1 -> PID Orig Boost/1(error)  "error"
  PID Orig Buck/1(Out1) -> Saturation1/1
  PID Orig Boost/1(Out1) -> Saturation/1

== system ACDCMG_woPV/Boost converter DC //CD 2 5 kHz - 300V /MPPT Controller using  "Incremental Conductance + Integral Regulator "  technique  ==
  note: +
  note: control mppt
  V_PV : Inport
  I_PV : Inport  Port=2
  Add : Sum  Inputs=+-
  Deblock MPPT : Step  Time=0.2  SampleTime=0
  Duty Cycle : Constant  Value=Dinit
  MPPT : Subsystem
  PWM Generator (DC-DC) : powerlib_meascontrol/Pulse & Signal Generators/PWM Generator (DC-DC)  Fsw=fc  Ts=Ts_Power
  Saturation : Saturate  UpperLimit=1  LowerLimit=0
  Pulses : Outport  VectorParamsAs1DForOutWhenUnconnected=off
  tag scope: D=global
  wires:
  V_PV/1 -> MPPT/1(V_PV)
  I_PV/1 -> MPPT/2(I_PV)
  PWM Generator (DC-DC)/1 -> Pulses/1
  Deblock MPPT/1 -> MPPT/3(on/off)
  Add/1 -> Saturation/1  "D"
  MPPT/1(Delta_D) -> Add/2  "Vdc_ref"
  Duty Cycle/1 -> Add/1
  Saturation/1 -> [D], PWM Generator (DC-DC)/1

== system ACDCMG_woPV/Boost converter DC //CD 2 5 kHz - 300V 1/MPPT Controller using  "Incremental Conductance + Integral Regulator "  technique  ==
  note: +
  note: control mppt
  V_PV : Inport
  I_PV : Inport  Port=2
  Add : Sum  Inputs=+-
  Deblock MPPT : Step  Time=0.2  SampleTime=0
  Duty Cycle : Constant  Value=Dinit
  MPPT : Subsystem
  PWM Generator (DC-DC) : powerlib_meascontrol/Pulse & Signal Generators/PWM Generator (DC-DC)  Fsw=fc  Ts=Ts_Power
  Saturation : Saturate  UpperLimit=1  LowerLimit=0
  Pulses : Outport  VectorParamsAs1DForOutWhenUnconnected=off
  tag scope: D=global
  wires:
  V_PV/1 -> MPPT/1(V_PV)
  I_PV/1 -> MPPT/2(I_PV)
  PWM Generator (DC-DC)/1 -> Pulses/1
  Deblock MPPT/1 -> MPPT/3(on/off)
  Add/1 -> Saturation/1  "D"
  MPPT/1(Delta_D) -> Add/2  "Vdc_ref"
  Duty Cycle/1 -> Add/1
  Saturation/1 -> [D], PWM Generator (DC-DC)/1

== system ACDCMG_woPV/Boost converter DC //DC 2 5 kHz - 300V /  ==
  V_PV : Inport
  I_PV : Inport  Port=2
  Duty Cycle : Constant  Value=0.34
  PWM Generator (DC-DC) : powerlib_meascontrol/Pulse & Signal Generators/PWM Generator (DC-DC)  Fsw=fc  Ts=Ts_Power
  Terminator1 : Terminator
  Terminator2 : Terminator
  Pulses : Outport  VectorParamsAs1DForOutWhenUnconnected=off
  tag scope: D=global
  wires:
  V_PV/1 -> Terminator1/1
  I_PV/1 -> Terminator2/1
  PWM Generator (DC-DC)/1 -> Pulses/1
  Duty Cycle/1 -> [D], PWM Generator (DC-DC)/1

== system ACDCMG_woPV/Bus_2/Power Factor Block1 ==
  Vabc : Inport
  Iabc : Inport  Port=2
  Complex to Magnitude-Angle : ComplexToMagnitudeAngle  Commented=on
  Conv pu1 : Gain  Gain=sqrt (3) /Vnom_sec  SaturateOnIntegerOverflow=on  OutDataTypeStr=Inherit: Same as input  ParamDataTypeStr=Inherit: Same as input
  Current3 : Goto  Commented=on  GotoTag=P_abc_Bus2  TagVisibility=global
  Current4 : Goto  Commented=on  GotoTag=Q_abc_Bus2  TagVisibility=global
  Mux : Mux  Inputs=2
  Power : spsPowerLib/Power  Commented=on  Freq=Freq  Vinit=Vinit  Iinit=Iinit  Ts=Ts
      settings: SourceProductBaseCode=PS
  Real-Imag to Complex : RealImagToComplex  Commented=on
  Terminator : Terminator  Commented=on
  cos(theta) : Trigonometry  Commented=on  Operator=cos
  to Kw : Gain  Commented=on  Gain=-1/1000
  to Kw1 : Gain  Commented=on  Gain=-1/1000
  "Vabc y Vabc " : Outport  VectorParamsAs1DForOutWhenUnconnected=off
  Iabc y Iabc : Outport  Port=2  VectorParamsAs1DForOutWhenUnconnected=off
  tag scope: Vabc_LL_pu_Bus2=global
  wires:
  Complex to Magnitude-Angle/2 -> cos(theta)/1
  Real-Imag to Complex/1 -> Complex to Magnitude-Angle/1
  cos(theta)/1 -> ?
  Complex to Magnitude-Angle/1 -> Terminator/1
  Iabc/1 -> Iabc y Iabc/1, Power/2
  Mux/1 -> "Vabc y Vabc "/1
  Vabc/1 -> Power/1, Conv pu1/1, Mux/1, Mux/2
  Conv pu1/1 -> [Vabc_LL_pu_Bus2]
  Power/1 -> to Kw1/1, Real-Imag to Complex/1
  Power/2 -> to Kw/1, Real-Imag to Complex/2
  to Kw/1 -> Current4/1
  to Kw1/1 -> Current3/1

== system ACDCMG_woPV/Bus_4/Power Factor Block1 ==
  Vabc : Inport
  Iabc : Inport  Port=2
  Complex to Magnitude-Angle : ComplexToMagnitudeAngle  Commented=on
  Conv pu1 : Gain  Gain=sqrt (3) /Vnom_sec  SaturateOnIntegerOverflow=on  OutDataTypeStr=Inherit: Same as input  ParamDataTypeStr=Inherit: Same as input
  Current3 : Goto  Commented=on  GotoTag=P_abc_Bus4  TagVisibility=global
  Current4 : Goto  Commented=on  GotoTag=Q_abc_Bus4  TagVisibility=global
  Mux : Mux  Inputs=2
  Power : spsPowerLib/Power  Commented=on  Freq=Freq  Vinit=Vinit  Iinit=Iinit  Ts=Ts
      settings: SourceProductBaseCode=PS
  Real-Imag to Complex : RealImagToComplex  Commented=on
  Terminator : Terminator  Commented=on
  cos(theta) : Trigonometry  Commented=on  Operator=cos
  to Kw : Gain  Commented=on  Gain=1/1000
  to Kw1 : Gain  Commented=on  Gain=1/1000
  Vabc y Vabc : Outport  VectorParamsAs1DForOutWhenUnconnected=off
  "Iabc y Iabc " : Outport  Port=2  VectorParamsAs1DForOutWhenUnconnected=off
  tag scope: Vabc_LL_pu_Bus4=global
  wires:
  Complex to Magnitude-Angle/2 -> cos(theta)/1
  Real-Imag to Complex/1 -> Complex to Magnitude-Angle/1
  cos(theta)/1 -> ?
  Complex to Magnitude-Angle/1 -> Terminator/1
  Iabc/1 -> "Iabc y Iabc "/1, Power/2
  Mux/1 -> Vabc y Vabc/1
  Conv pu1/1 -> [Vabc_LL_pu_Bus4]
  Vabc/1 -> Power/1, Conv pu1/1, Mux/1, Mux/2
  Power/2 -> Real-Imag to Complex/2, to Kw/1
  Power/1 -> to Kw1/1, Real-Imag to Complex/1
  to Kw/1 -> Current4/1
  to Kw1/1 -> Current3/1

== system ACDCMG_woPV/Bus_5/Power Factor Block1 ==
  Vabc : Inport
  Iabc : Inport  Port=2
  Complex to Magnitude-Angle : ComplexToMagnitudeAngle  Commented=on
  Conv pu1 : Gain  Gain=sqrt (3) /Vnom_sec  SaturateOnIntegerOverflow=on  OutDataTypeStr=Inherit: Same as input  ParamDataTypeStr=Inherit: Same as input
  Current3 : Goto  Commented=on  GotoTag=P_abc_Bus5  TagVisibility=global
  Current4 : Goto  Commented=on  GotoTag=Q_abc_Bus5  TagVisibility=global
  Mux : Mux  Inputs=2
  Power : spsPowerLib/Power  Commented=on  Freq=Freq  Vinit=Vinit  Iinit=Iinit  Ts=Ts
      settings: SourceProductBaseCode=PS
  Real-Imag to Complex : RealImagToComplex  Commented=on
  Terminator : Terminator  Commented=on
  cos(theta) : Trigonometry  Commented=on  Operator=cos
  to Kw : Gain  Commented=on  Gain=1/1000
  to Kw1 : Gain  Commented=on  Gain=1/1000
  Vabc y Vabc : Outport  VectorParamsAs1DForOutWhenUnconnected=off
  "Iabc y Iabc " : Outport  Port=2  VectorParamsAs1DForOutWhenUnconnected=off
  tag scope: Vabc_LL_pu_Bus5=global
  wires:
  Complex to Magnitude-Angle/2 -> cos(theta)/1
  Real-Imag to Complex/1 -> Complex to Magnitude-Angle/1
  cos(theta)/1 -> ?
  Complex to Magnitude-Angle/1 -> Terminator/1
  Iabc/1 -> "Iabc y Iabc "/1, Power/2
  Mux/1 -> Vabc y Vabc/1
  Conv pu1/1 -> [Vabc_LL_pu_Bus5]
  Vabc/1 -> Power/1, Conv pu1/1, Mux/1, Mux/2
  Power/2 -> Real-Imag to Complex/2, to Kw/1
  Power/1 -> to Kw1/1, Real-Imag to Complex/1
  to Kw/1 -> Current4/1
  to Kw1/1 -> Current3/1

== system ACDCMG_woPV/Bus_7/Power Factor Block1 ==
  Vabc : Inport
  Iabc : Inport  Port=2
  Complex to Magnitude-Angle : ComplexToMagnitudeAngle  Commented=on
  Conv pu2 : Gain  Gain=sqrt (3) /Vnom_prim  SaturateOnIntegerOverflow=on  OutDataTypeStr=Inherit: Same as input  ParamDataTypeStr=Inherit: Same as input
  Current3 : Goto  Commented=on  GotoTag=P_abc_Bus7  TagVisibility=global
  Current4 : Goto  Commented=on  GotoTag=Q_abc_Bus7  TagVisibility=global
  Mux : Mux  Inputs=2
  Power : spsPowerLib/Power  Commented=on  Freq=Freq  Vinit=Vinit  Iinit=Iinit  Ts=Ts
      settings: SourceProductBaseCode=PS
  Real-Imag to Complex : RealImagToComplex  Commented=on
  Terminator : Terminator  Commented=on
  cos(theta) : Trigonometry  Commented=on  Operator=cos
  to Kw : Gain  Commented=on  Gain=1/1000
  to Kw1 : Gain  Commented=on  Gain=1/1000
  "Vabc y Vabc " : Outport  VectorParamsAs1DForOutWhenUnconnected=off
  "Iabc y Iabc " : Outport  Port=2  VectorParamsAs1DForOutWhenUnconnected=off
  tag scope: Vabc_LL_pu_Bus7=global
  wires:
  Complex to Magnitude-Angle/2 -> cos(theta)/1
  Real-Imag to Complex/1 -> Complex to Magnitude-Angle/1
  cos(theta)/1 -> ?
  Complex to Magnitude-Angle/1 -> Terminator/1
  Iabc/1 -> "Iabc y Iabc "/1, Power/2
  Mux/1 -> "Vabc y Vabc "/1
  Conv pu2/1 -> [Vabc_LL_pu_Bus7]
  Vabc/1 -> Power/1, Conv pu2/1, Mux/1, Mux/2
  Power/2 -> Real-Imag to Complex/2, to Kw/1
  Power/1 -> to Kw1/1, Real-Imag to Complex/1
  to Kw/1 -> Current4/1
  to Kw1/1 -> Current3/1

== system ACDCMG_woPV/Bus_8      /Power Factor Block1 ==
  Vabc : Inport
  Iabc : Inport  Port=2
  Complex to Magnitude-Angle : ComplexToMagnitudeAngle  Commented=on
  Conv pu2 : Gain  Gain=sqrt (3) /Vnom_Diesel  SaturateOnIntegerOverflow=on  OutDataTypeStr=Inherit: Same as input  ParamDataTypeStr=Inherit: Same as input
  Current3 : Goto  Commented=on  GotoTag=P_abc_Bus8  TagVisibility=global
  Current4 : Goto  Commented=on  GotoTag=Q_abc_Bus8  TagVisibility=global
  Gain : Gain  Commented=on  Gain=-1/1000
  Gain1 : Gain  Commented=on  Gain=-1/1000
  Mux : Mux  Inputs=2
  Power : spsPowerLib/Power  Commented=on  Freq=Freq  Vinit=Vinit  Iinit=Iinit  Ts=Ts
      settings: SourceProductBaseCode=PS
  Real-Imag to Complex : RealImagToComplex  Commented=on
  Terminator : Terminator  Commented=on
  cos(theta) : Trigonometry  Commented=on  Operator=cos
  "Vabc y Vabc " : Outport  VectorParamsAs1DForOutWhenUnconnected=off
  "Iabc y Iabc " : Outport  Port=2  VectorParamsAs1DForOutWhenUnconnected=off
  tag scope: Vabc_LL_pu_Bus8=global
  wires:
  Complex to Magnitude-Angle/2 -> cos(theta)/1
  Real-Imag to Complex/1 -> Complex to Magnitude-Angle/1
  cos(theta)/1 -> ?
  Complex to Magnitude-Angle/1 -> Terminator/1
  Iabc/1 -> "Iabc y Iabc "/1, Power/2
  Mux/1 -> "Vabc y Vabc "/1
  Conv pu2/1 -> [Vabc_LL_pu_Bus8]
  Vabc/1 -> Power/1, Conv pu2/1, Mux/1, Mux/2
  Power/2 -> Real-Imag to Complex/2, Gain/1
  Power/1 -> Gain1/1, Real-Imag to Complex/1
  Gain/1 -> Current4/1
  Gain1/1 -> Current3/1

== system ACDCMG_woPV/Bus_AC//DC3/Battery system ==
  note: DC Bus
  note: Bettery
  "0 = Enable (Do it after transient, so that it does not calculate ripples during transient) 1 = Reset after every change in current reference" : Constant  Value=0
  Current Inst : Scope
  Current going to/ from the battery : Scope
  Display6 : Display
  Mean : spsMeanLib/Mean  Freq=10  Vinit=0  Ts=0
  Power : Product
  Power Bess : Scope
  Ripple Calculations : Subsystem
  Ripple in Boost : Display
  Ripple in Buck : Display
  Vbat : Scope
  Vdc : Scope
  to Kw : Gain  Gain=1/1000
  wires:
  to Kw/1 -> Display6/1, Power Bess/1
  Mean/1 -> Power/2
  Power/1 -> to Kw/1
  Ripple Calculations/1(Ripple in Buck) -> Ripple in Buck/1
  "0 = Enable (Do it after transient, so that it does not calculate ripples during transient) 1 = Reset after every change in current reference"/1 -> Ripple Calculations/2(Reset)
  Ripple Calculations/2(Ripple in Boost) -> Ripple in Boost/1
  [Idc_bus] -> Mean/1, Ripple Calculations/1(Signal), Current Inst/1
  [current] -> Current going to/ from the battery/1
  [Vdc_bus] -> Vdc/1, Power/1
  [Vdc_battery] -> Vbat/1

== system ACDCMG_woPV/Bus_AC//DC3/PV system ==
  note: Bus DC
  note: PV
  Bus Selector : BusSelector  OutputSignals=V_PV,I_PV,I_diode,Irradiance (W/m2),Temperature (deg C)
  Current going to/ DC bus : Scope
  "P (kW) " : Display
      settings: Format=bank  Decimation=2000
  PV : Scope  NumInputPorts=3
  PV1 : Scope  NumInputPorts=5
  Pmean : Subsystem
  Vdc Boost : Display
      settings: Format=bank  Decimation=2000
  Vdc DC bus : Scope
  tag scope: I_PV=global, Idiode_PV=global, Ir=global, Temp=global, V_PV=global
  wires:
  [V_PV] -> PV/1  "V_PV"
  [I_PV] -> PV/2  "I_PV"
  [Idiode_PV] -> PV/3  "Idiode_PV"
  [m_PV] -> Bus Selector/1
  Bus Selector/1 -> [V_PV]  "<V_PV>"
  Bus Selector/2 -> [I_PV]  "<I_PV>"
  Bus Selector/4 -> [Ir]  "<Irradiance (W/m2)>"
  Bus Selector/3 -> [Idiode_PV]  "<I_diode>"
  Bus Selector/5 -> [Temp]  "<Temperature (deg C)>"
  [Temp] -> PV1/2  "Temp (deg. C)"
  [D] -> PV1/5  "Duty Cycle"
  Pmean/2(V) -> Vdc Boost/1, PV1/4  "Vmean (V)"
  [Ir] -> PV1/1  "Ir (W/m^2)"
  Pmean/1(P) -> "P (kW) "/1, PV1/3  "Pmean  (kW)"
  [I_DC_bus_PV] -> Current going to/ DC bus/1
  [V_DC_bus_PV] -> Vdc DC bus/1

== system ACDCMG_woPV/Bus_AC//DC4/Power Factor Block1 ==
  Vabc : Inport
  Iabc : Inport  Port=2
  Complex to Magnitude-Angle : ComplexToMagnitudeAngle  Commented=on
  Power : spsPowerLib/Power  Commented=on  Freq=Freq  Vinit=Vinit  Iinit=Iinit  Ts=Ts
      settings: SourceProductBaseCode=PS
  Real-Imag to Complex : RealImagToComplex  Commented=on
  Terminator : Terminator  Commented=on
  cos(theta) : Trigonometry  Commented=on  Operator=cos
  "Vabc y Vabc " : Outport  VectorParamsAs1DForOutWhenUnconnected=off
  "Iabc y Iabc " : Outport  Port=2  VectorParamsAs1DForOutWhenUnconnected=off
  wires:
  Power/1 -> Real-Imag to Complex/1
  Power/2 -> Real-Imag to Complex/2
  Complex to Magnitude-Angle/2 -> cos(theta)/1
  Real-Imag to Complex/1 -> Complex to Magnitude-Angle/1
  cos(theta)/1 -> ?
  Complex to Magnitude-Angle/1 -> Terminator/1
  Iabc/1 -> "Iabc y Iabc "/1, Power/2
  Vabc/1 -> "Vabc y Vabc "/1, Power/1

== system ACDCMG_woPV/Bus_AC//DC5/Power Factor Block1 ==
  Vabc : Inport
  Iabc : Inport  Port=2
  Complex to Magnitude-Angle : ComplexToMagnitudeAngle
  Power : spsPowerLib/Power  Freq=Freq  Vinit=Vinit  Iinit=Iinit  Ts=Ts
      settings: SourceProductBaseCode=PS
  Real-Imag to Complex : RealImagToComplex
  Terminator : Terminator
  cos(theta) : Trigonometry  Operator=cos
  "Vabc y Vabc " : Outport  VectorParamsAs1DForOutWhenUnconnected=off
  "Iabc y Iabc " : Outport  Port=2  VectorParamsAs1DForOutWhenUnconnected=off
  Outport : Outport  Port=3
  wires:
  Power/1 -> Real-Imag to Complex/1
  Power/2 -> Real-Imag to Complex/2
  Complex to Magnitude-Angle/2 -> cos(theta)/1
  Real-Imag to Complex/1 -> Complex to Magnitude-Angle/1
  cos(theta)/1 -> Outport/1
  Complex to Magnitude-Angle/1 -> Terminator/1
  Iabc/1 -> "Iabc y Iabc "/1, Power/2
  Vabc/1 -> Power/1, "Vabc y Vabc "/1

== system ACDCMG_woPV/DATA  ADQUISITION/Power_Losses_abc ==
  From10 : From  Commented=on  GotoTag=Power_Losse_abc_L10  TagVisibility=global
  From11 : From  Commented=on  GotoTag=Power_Losse_abc_L10
  From12 : From  Commented=on  GotoTag=Power_Losse_abc_L12
  From13 : From  Commented=on  GotoTag=Power_Losse_abc_L14
  From6 : From  Commented=on  GotoTag=Power_Losse_abc_L3  TagVisibility=global
  Mux : Mux  Inputs=9
  f2 : ToWorkspace  VariableName=Power_Losse_abc  SaveFormat=Timeseries  SampleTime=-1
  wires:
  [Power_Losse_abc_L1] -> Mux/1
  Mux/1 -> f2/1
  [Power_Losse_abc_L2] -> Mux/2
  [Power_Losse_abc_L5] -> Mux/5
  [Power_Losse_abc_L6] -> Mux/6
  [Power_Losse_abc_L7] -> Mux/7
  [Power_Losse_abc_L3] -> Mux/3
  [Power_Losse_abc_L4] -> Mux/4
  [Power_Losse_abc_L8] -> Mux/8
  [Power_Losse_abc_L9] -> Mux/9

== system ACDCMG_woPV/DATA  ADQUISITION/VoltageLL_pu_abc ==
  From28 : From  Commented=on  GotoTag=Vabc_LL_pu_Bus10
  From31 : From  Commented=on  GotoTag=Vabc_LL_pu_Bus10
  From34 : From  Commented=on  GotoTag=Vabc_LL_pu_Bus12
  From40 : From  Commented=on  GotoTag=Vabc_LL_pu_Bus14
  Mux : Mux  Inputs=10
  f2 : ToWorkspace  VariableName=VoltageLL_pu_abc  SaveFormat=Timeseries  SampleTime=-1
  wires:
  [Vabc_LL_pu_Bus4] -> Mux/4
  [Vabc_LL_pu_Bus5] -> Mux/5
  Mux/1 -> f2/1
  [Vabc_LL_pu_Bus8] -> Mux/8
  [Vabc_LL_pu_Bus1] -> Mux/1
  [Vabc_LL_pu_Bus2] -> Mux/2
  [Vabc_LL_pu_Bus6] -> Mux/6
  [Vabc_LL_pu_Bus7] -> Mux/7
  [V_pu_BusDC] -> Mux/10
  [Vabc_LL_pu_Bus3] -> Mux/3
  [Vabc_LL_pu_Bus9] -> Mux/9
